simulink model "gm_uz_inverter_status"  (R2024a)
settings: Solver=FixedStepDiscrete  StartTime=0.0  StopTime=100e-6  RelTol=1e-3  EnableMultiTasking=on
libraries: hdlsllib x16
settings Model: Creator=Geiger  LastModifiedBy=Geiger
settings SolverCC: PositivePriorityOrder=on
settings OptimizationCC: BlockReduction=off  ConditionallyExecuteInputs=off  DefaultParameterBehavior=Inlined  EnhancedBackFolding=on  PassReuseOutputArgsAs=Individual arguments  ZeroExternalMemoryAtStartup=off  ZeroInternalMemoryAtStartup=off  MaxStackSize=64  OptimizeBlockOrder=speed  DifferentSizesBufferReuse=on  OptimizationCustomize=off  EfficientTunableParamExpr=on
settings DebuggingCC: AlgebraicLoopMsg=error  InheritedTsInSrcMsg=none  ParameterTunabilityLossMsg=error
settings HardwareCC: ProdBitPerPointer=32  ProdBitPerSizeT=32  ProdBitPerPtrDiffT=32  ProdLargestAtomicFloat=None  ProdIntDivRoundTo=Undefined  ProdEndianess=Unspecified  ProdWordSize=32  ProdHWDeviceType=ASIC/FPGA->ASIC/FPGA  TargetBitPerPointer=64  TargetBitPerSizeT=64  TargetBitPerPtrDiffT=64  TargetLongLongMode=on  TargetIntDivRoundTo=Zero  TargetEndianess=LittleEndian  TargetWordSize=64  TargetHWDeviceType=Custom Processor->MATLAB Host Computer  ProdEqTarget=off
settings ModelReferenceCC: EnableRefExpFcnMdlSchedulingChecks=on
settings SFSimCC: MATLABDynamicMemAlloc=off
settings RTWCC: Description=Embedded Coder  SystemTargetFile=ert.tlc  TemplateMakefile=ert_default_tmf  Toolchain=Linaro AArch64 Linux v6.3.1
settings CodeAppCC: ForceParamTrailComments=on  IgnoreCustomStorageClasses=off  OperatorAnnotations=on  SimulinkDataObjDesc=on  SFDataObjDesc=on  InsertBlockDesc=on
settings ERTTargetCC: InlinedParameterPlacement=NonHierarchical  ERTCustomFileTemplate=example_file_process.tlc

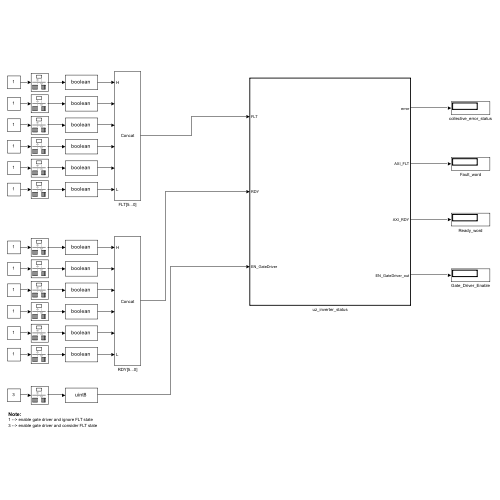
[thumbnail: Simulink's stored preview of the top-level diagram]
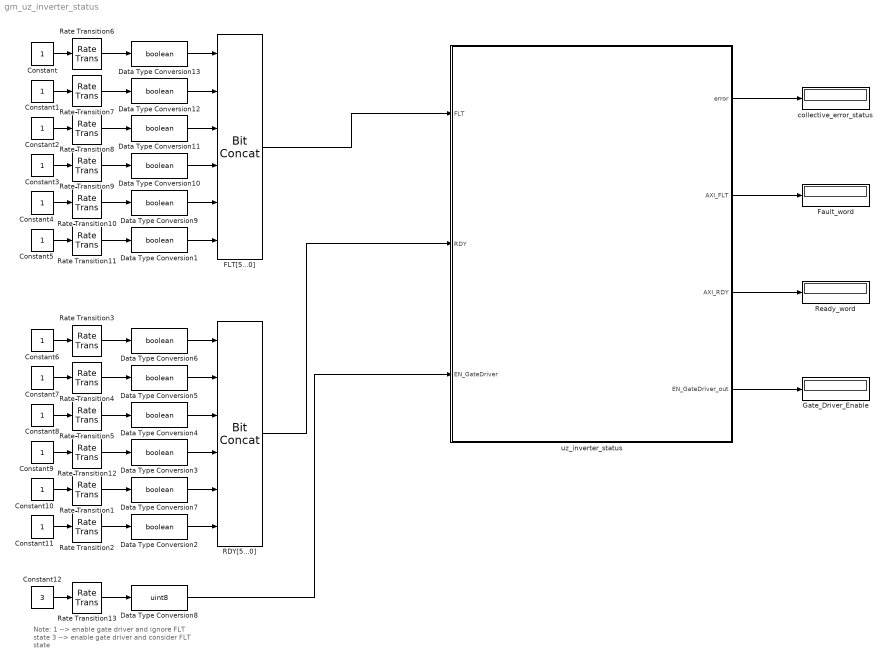
== system gm_uz_inverter_status ==
  note: Note:
      | 1 --> enable gate driver and ignore FLT state
      | 3 --> enable gate driver and consider FLT state
  Constant{,1..11} (12 alike) : Constant
  Constant12 : Constant  Value=3
  Data Type Conversion{1..7,9..13} (12 alike) : DataTypeConversion  OutDataTypeStr=boolean  SaturateOnIntegerOverflow=off  RndMeth=Floor
  Data Type Conversion8 : DataTypeConversion  OutDataTypeStr=uint8  SaturateOnIntegerOverflow=off  RndMeth=Floor
  FLT[5...0] : hdlsllib/Logic and Bit Operations/Bit Concat  numInputs=6
  Fault_word : Display
      settings: Format=binary (Stored Integer)
  Gate_Driver_Enable : Display
      settings: Format=binary (Stored Integer)
  RDY[5...0] : hdlsllib/Logic and Bit Operations/Bit Concat  numInputs=6
  Rate Transition{1..13} (13 alike) : RateTransition  OutPortSampleTime=t_clk
  Ready_word : Display
      settings: Format=binary (Stored Integer)
  collective_error_status : Display
  uz_inverter_status : Subsystem  TreatAsAtomicUnit=on
  wires:
  Data Type Conversion8/1 -> uz_inverter_status/3(EN_GateDriver)
  Rate Transition13/1 -> Data Type Conversion8/1
  Constant12/1 -> Rate Transition13/1
  uz_inverter_status/4(EN_GateDriver_out) -> Gate_Driver_Enable/1
  uz_inverter_status/1(error) -> collective_error_status/1
  uz_inverter_status/3(AXI_RDY) -> Ready_word/1
  uz_inverter_status/2(AXI_FLT) -> Fault_word/1
  Rate Transition2/1 -> Data Type Conversion2/1
  RDY[5...0]/1 -> uz_inverter_status/2(RDY)
  Constant8/1 -> Rate Transition5/1
  Constant7/1 -> Rate Transition4/1
  Data Type Conversion2/1 -> RDY[5...0]/6
  Rate Transition4/1 -> Data Type Conversion5/1
  Rate Transition1/1 -> Data Type Conversion7/1
  Rate Transition3/1 -> Data Type Conversion6/1
  Rate Transition12/1 -> Data Type Conversion3/1
  Data Type Conversion5/1 -> RDY[5...0]/2
  Data Type Conversion3/1 -> RDY[5...0]/4
  Data Type Conversion6/1 -> RDY[5...0]/1
  Rate Transition5/1 -> Data Type Conversion4/1
  Constant10/1 -> Rate Transition1/1
  Data Type Conversion4/1 -> RDY[5...0]/3
  Constant11/1 -> Rate Transition2/1
  Constant9/1 -> Rate Transition12/1
  Constant6/1 -> Rate Transition3/1
  Data Type Conversion7/1 -> RDY[5...0]/5
  Data Type Conversion11/1 -> FLT[5...0]/3
  Constant/1 -> Rate Transition6/1
  Constant3/1 -> Rate Transition9/1
  Constant5/1 -> Rate Transition11/1
  Rate Transition8/1 -> Data Type Conversion11/1
  Constant2/1 -> Rate Transition8/1
  Constant4/1 -> Rate Transition10/1
  Constant1/1 -> Rate Transition7/1
  Data Type Conversion13/1 -> FLT[5...0]/1
  Data Type Conversion9/1 -> FLT[5...0]/5
  Rate Transition9/1 -> Data Type Conversion10/1
  Data Type Conversion10/1 -> FLT[5...0]/4
  Data Type Conversion12/1 -> FLT[5...0]/2
  Data Type Conversion1/1 -> FLT[5...0]/6
  Rate Transition7/1 -> Data Type Conversion12/1
  Rate Transition6/1 -> Data Type Conversion13/1
  Rate Transition10/1 -> Data Type Conversion9/1
  FLT[5...0]/1 -> uz_inverter_status/1(FLT)
  Rate Transition11/1 -> Data Type Conversion1/1

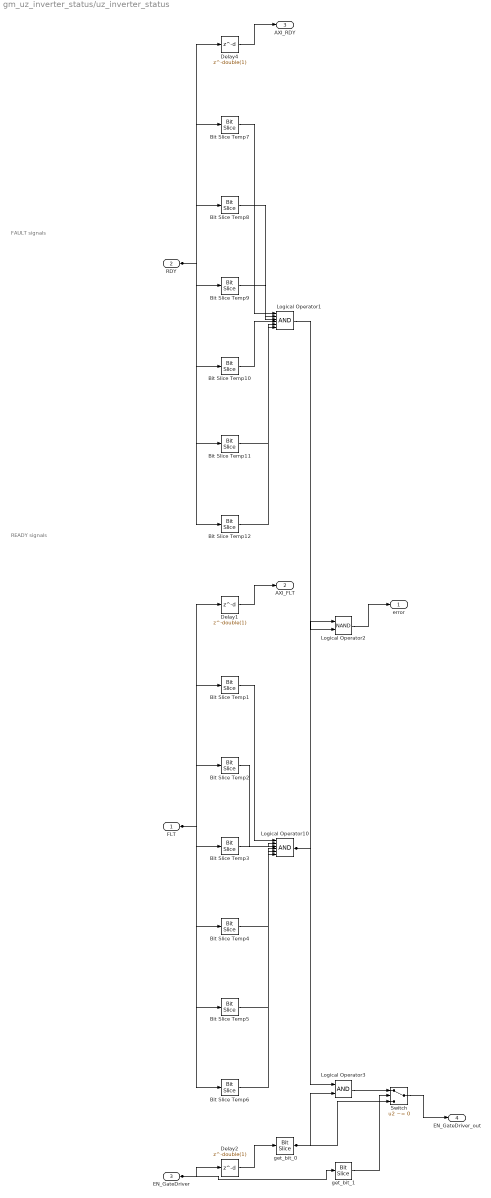
== system gm_uz_inverter_status/uz_inverter_status ==
  note: READY signals
  note: FAULT signals
  FLT : Inport  OutDataTypeStr=fixdt(0, 6, 0)  PortDimensions=1  SampleTime=1e-08
  RDY : Inport  Port=2  OutDataTypeStr=fixdt(0, 6, 0)  PortDimensions=1  SampleTime=1e-08
  EN_GateDriver : Inport  Port=3  OutDataTypeStr=uint8  PortDimensions=1  SampleTime=1e-08
  Bit Slice Temp1 : hdlsllib/Logic and Bit Operations/Bit Slice  lidx=double(0)  ridx=double(0)
  Bit Slice Temp10 : hdlsllib/Logic and Bit Operations/Bit Slice  lidx=double(3)  ridx=double(3)
  Bit Slice Temp11 : hdlsllib/Logic and Bit Operations/Bit Slice  lidx=double(4)  ridx=double(4)
  Bit Slice Temp12 : hdlsllib/Logic and Bit Operations/Bit Slice  lidx=double(5)  ridx=double(5)
  Bit Slice Temp2 : hdlsllib/Logic and Bit Operations/Bit Slice  lidx=double(1)  ridx=double(1)
  Bit Slice Temp3 : hdlsllib/Logic and Bit Operations/Bit Slice  lidx=double(2)  ridx=double(2)
  Bit Slice Temp4 : hdlsllib/Logic and Bit Operations/Bit Slice  lidx=double(3)  ridx=double(3)
  Bit Slice Temp5 : hdlsllib/Logic and Bit Operations/Bit Slice  lidx=double(4)  ridx=double(4)
  Bit Slice Temp6 : hdlsllib/Logic and Bit Operations/Bit Slice  lidx=double(5)  ridx=double(5)
  Bit Slice Temp7 : hdlsllib/Logic and Bit Operations/Bit Slice  lidx=double(0)  ridx=double(0)
  Bit Slice Temp8 : hdlsllib/Logic and Bit Operations/Bit Slice  lidx=double(1)  ridx=double(1)
  Bit Slice Temp9 : hdlsllib/Logic and Bit Operations/Bit Slice  lidx=double(2)  ridx=double(2)
  Delay1 : Delay  DelayLength=double(1)  InitialCondition=0  SampleTime=1e-08
  Delay2 : Delay  DelayLength=double(1)  InitialCondition=0  SampleTime=1e-08
  Delay4 : Delay  DelayLength=double(1)  InitialCondition=0  SampleTime=1e-08
  Logical Operator1 : Logic  Inputs=6  AllPortsSameDT=off  OutDataTypeStr=boolean  SampleTime=1e-08
  Logical Operator10 : Logic  Inputs=6  AllPortsSameDT=off  OutDataTypeStr=boolean  SampleTime=1e-08
  Logical Operator2 : Logic  Operator=NAND  AllPortsSameDT=off  OutDataTypeStr=boolean  SampleTime=1e-08
  Logical Operator3 : Logic  AllPortsSameDT=off  OutDataTypeStr=boolean  SampleTime=1e-08
  Switch : Switch  Criteria=u2 ~= 0  Threshold=double(0)  OutDataTypeStr=boolean  SampleTime=1e-08  SaturateOnIntegerOverflow=off  InputSameDT=off
  get_bit_0 : hdlsllib/Logic and Bit Operations/Bit Slice  lidx=double(0)  ridx=double(0)
  get_bit_1 : hdlsllib/Logic and Bit Operations/Bit Slice  lidx=double(1)  ridx=double(1)
  error : Outport  SampleTime=1e-08  VectorParamsAs1DForOutWhenUnconnected=off
  AXI_FLT : Outport  Port=2  PortDimensions=1  SampleTime=1e-08  VectorParamsAs1DForOutWhenUnconnected=off
  AXI_RDY : Outport  Port=3  PortDimensions=1  SampleTime=1e-08  VectorParamsAs1DForOutWhenUnconnected=off
  EN_GateDriver_out : Outport  Port=4  SampleTime=1e-08  VectorParamsAs1DForOutWhenUnconnected=off
  wires:
  FLT/1 -> Bit Slice Temp6/1, Bit Slice Temp5/1, Bit Slice Temp4/1, Bit Slice Temp3/1, Bit Slice Temp2/1, Bit Slice Temp1/1, Delay1/1
  RDY/1 -> Bit Slice Temp9/1, Bit Slice Temp8/1, Bit Slice Temp7/1, Bit Slice Temp12/1, Bit Slice Temp11/1, Bit Slice Temp10/1, Delay4/1
  EN_GateDriver/1 -> get_bit_1/1, Delay2/1
  Bit Slice Temp1/1 -> Logical Operator10/1
  Bit Slice Temp10/1 -> Logical Operator1/4
  Bit Slice Temp11/1 -> Logical Operator1/5
  Bit Slice Temp12/1 -> Logical Operator1/6
  Bit Slice Temp2/1 -> Logical Operator10/2
  Bit Slice Temp3/1 -> Logical Operator10/3
  Bit Slice Temp4/1 -> Logical Operator10/4
  Bit Slice Temp5/1 -> Logical Operator10/5
  Bit Slice Temp6/1 -> Logical Operator10/6
  Bit Slice Temp7/1 -> Logical Operator1/1
  Bit Slice Temp8/1 -> Logical Operator1/2
  Bit Slice Temp9/1 -> Logical Operator1/3
  Delay1/1 -> AXI_FLT/1
  Delay2/1 -> get_bit_0/1
  Delay4/1 -> AXI_RDY/1
  Logical Operator1/1 -> Logical Operator2/2
  Logical Operator10/1 -> Logical Operator3/1, Logical Operator2/1
  Logical Operator2/1 -> error/1
  Logical Operator3/1 -> Switch/1
  Switch/1 -> EN_GateDriver_out/1
  get_bit_0/1 -> Switch/3, Logical Operator3/2
  get_bit_1/1 -> Switch/2
